simulink model "Tclab_simulink_model"  (R2021a)
settings: Solver=VariableStepAuto  StartTime=0.0  StopTime=600  RelTol=1e-3
undefined symbols (not defined in the file or in its folder): DiscIntNeverNeededParam, Discrete, ee_sli_rtmsupport, gcbh, Time
libraries: realtime_pacer_lib x2, sharedTrackingLibrary x1, ctrlSharedLib x1
settings Model: Creator=Arman  LastModifiedBy=Arman

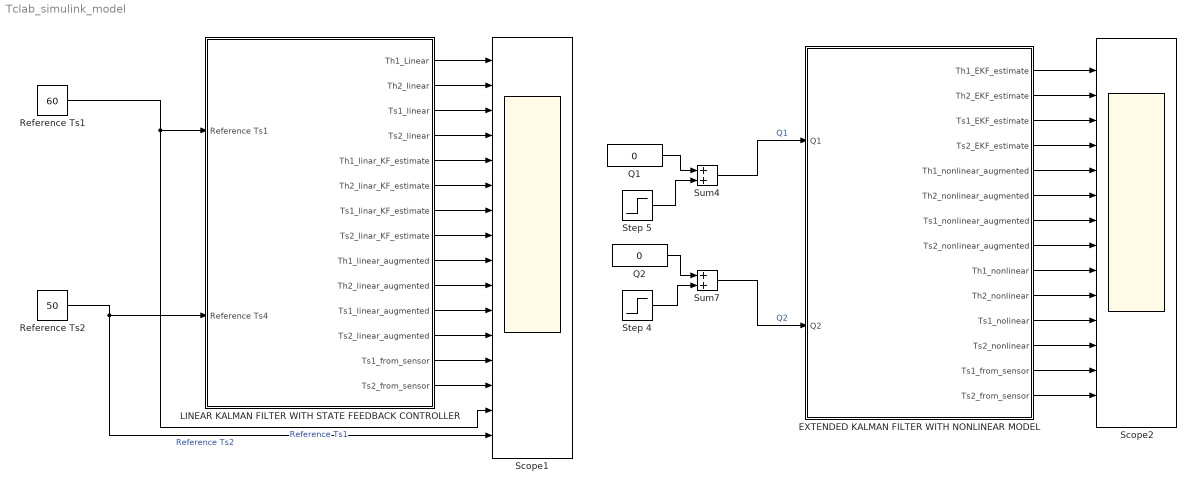
== system Tclab_simulink_model ==
  EXTENDED KALMAN FILTER WITH NONLINEAR MODEL : Subsystem
  LINEAR KALMAN FILTER WITH STATE FEEDBACK CONTROLLER : Subsystem
  Q1 : Constant  Value=0  SampleTime=1
  Q2 : Constant  Value=0  SampleTime=1
  "Reference Ts1 " : Constant  Value=60  SampleTime=1
  Reference Ts2 : Constant  Value=50  SampleTime=1
  Scope1 : Scope  NumInputPorts=16
  Scope2 : Scope  NumInputPorts=14
  Step 4 : Step  Time=300  Before=80  After=0  SampleTime=1
  Step 5 : Step  Time=300  After=80  SampleTime=1
  Sum4 : Sum  InputSameDT=on  SaturateOnIntegerOverflow=on  OutDataTypeStr=Inherit: Same as first input
  Sum7 : Sum  InputSameDT=on  SaturateOnIntegerOverflow=on  OutDataTypeStr=Inherit: Same as first input
  wires:
  "Reference Ts1 "/1 -> LINEAR KALMAN FILTER WITH STATE FEEDBACK CONTROLLER/1(Reference Ts1), Scope1/15  "Reference Ts1"
  Reference Ts2/1 -> Scope1/16, LINEAR KALMAN FILTER WITH STATE FEEDBACK CONTROLLER/2(Reference Ts4)  "Reference Ts2"
  Step 4/1 -> Sum7/2
  Q2/1 -> Sum7/1
  Step 5/1 -> Sum4/2
  Q1/1 -> Sum4/1
  Sum4/1 -> EXTENDED KALMAN FILTER WITH NONLINEAR MODEL/1(Q1)  "Q1"
  Sum7/1 -> EXTENDED KALMAN FILTER WITH NONLINEAR MODEL/2(Q2)  "Q2"
  LINEAR KALMAN FILTER WITH STATE FEEDBACK CONTROLLER/1(Th1_Linear) -> Scope1/1
  LINEAR KALMAN FILTER WITH STATE FEEDBACK CONTROLLER/2(Th2_linear) -> Scope1/2
  LINEAR KALMAN FILTER WITH STATE FEEDBACK CONTROLLER/3(Ts1_linear) -> Scope1/3
  LINEAR KALMAN FILTER WITH STATE FEEDBACK CONTROLLER/4(Ts2_linear) -> Scope1/4
  LINEAR KALMAN FILTER WITH STATE FEEDBACK CONTROLLER/5(Th1_linar_KF_estimate) -> Scope1/5
  LINEAR KALMAN FILTER WITH STATE FEEDBACK CONTROLLER/6(Th2_linar_KF_estimate) -> Scope1/6
  LINEAR KALMAN FILTER WITH STATE FEEDBACK CONTROLLER/7(Ts1_linar_KF_estimate) -> Scope1/7
  LINEAR KALMAN FILTER WITH STATE FEEDBACK CONTROLLER/8(Ts2_linar_KF_estimate) -> Scope1/8
  LINEAR KALMAN FILTER WITH STATE FEEDBACK CONTROLLER/9(Th1_linear_augmented) -> Scope1/9
  LINEAR KALMAN FILTER WITH STATE FEEDBACK CONTROLLER/10(Th2_linear_augmented) -> Scope1/10
  LINEAR KALMAN FILTER WITH STATE FEEDBACK CONTROLLER/11(Ts1_linear_augmented) -> Scope1/11
  LINEAR KALMAN FILTER WITH STATE FEEDBACK CONTROLLER/12(Ts2_linear_augmented) -> Scope1/12
  LINEAR KALMAN FILTER WITH STATE FEEDBACK CONTROLLER/13(Ts1_from_sensor) -> Scope1/13
  LINEAR KALMAN FILTER WITH STATE FEEDBACK CONTROLLER/14(Ts2_from_sensor) -> Scope1/14
  EXTENDED KALMAN FILTER WITH NONLINEAR MODEL/1(Th1_EKF_estimate) -> Scope2/1
  EXTENDED KALMAN FILTER WITH NONLINEAR MODEL/2(Th2_EKF_estimate) -> Scope2/2
  EXTENDED KALMAN FILTER WITH NONLINEAR MODEL/3(Ts1_EKF_estimate) -> Scope2/3
  EXTENDED KALMAN FILTER WITH NONLINEAR MODEL/4(Ts2_EKF_estimate) -> Scope2/4
  EXTENDED KALMAN FILTER WITH NONLINEAR MODEL/5(Th1_nonlinear_augmented) -> Scope2/5
  EXTENDED KALMAN FILTER WITH NONLINEAR MODEL/6(Th2_nonlinear_augmented) -> Scope2/6
  EXTENDED KALMAN FILTER WITH NONLINEAR MODEL/7(Ts1_nonlinear_augmented) -> Scope2/7
  EXTENDED KALMAN FILTER WITH NONLINEAR MODEL/8(Ts2_nonlinear_augmented) -> Scope2/8
  EXTENDED KALMAN FILTER WITH NONLINEAR MODEL/9(Th1_nonlinear) -> Scope2/9
  EXTENDED KALMAN FILTER WITH NONLINEAR MODEL/10(Th2_nonlinear) -> Scope2/10
  EXTENDED KALMAN FILTER WITH NONLINEAR MODEL/11(Ts1_nolinear) -> Scope2/11
  EXTENDED KALMAN FILTER WITH NONLINEAR MODEL/12(Ts2_nonlinear) -> Scope2/12
  EXTENDED KALMAN FILTER WITH NONLINEAR MODEL/13(Ts1_from_sensor) -> Scope2/13
  EXTENDED KALMAN FILTER WITH NONLINEAR MODEL/14(Ts2_from_sensor) -> Scope2/14

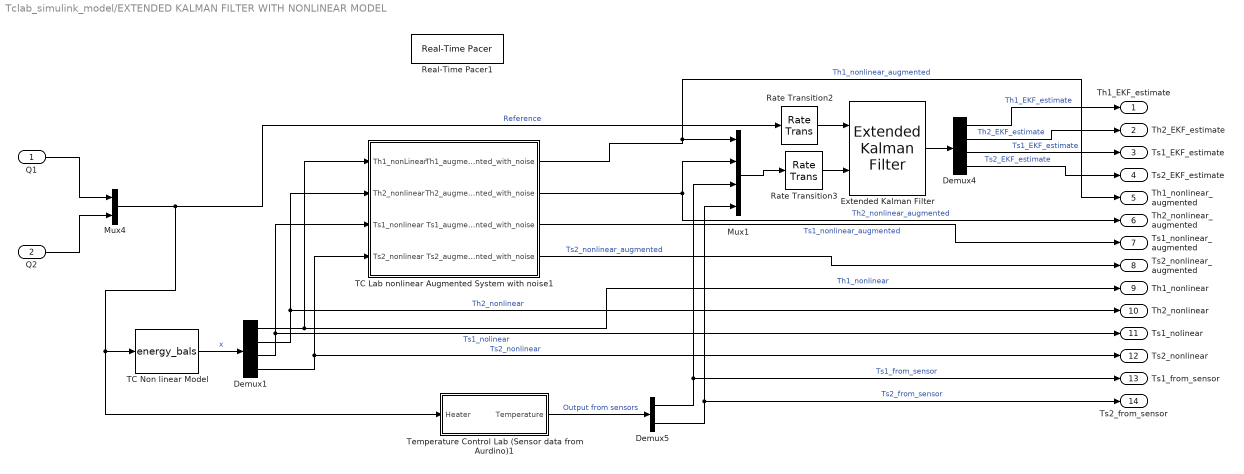
== system Tclab_simulink_model/EXTENDED KALMAN FILTER WITH NONLINEAR MODEL ==
  Q1 : Inport
  Q2 : Inport  Port=2
  Demux1 : Demux  Outputs=[1,1,1,1]
  Demux4 : Demux  Outputs=[1,1,1,1]
  Demux5 : Demux  Outputs=2
  Extended Kalman Filter : sharedTrackingLibrary/Extended Kalman Filter  StateTransitionFcn=myStateTransitionFcn  HasStateTransitionJacobianFcn=off  HasAdditiveProcessNoise=Additive  ProcessNoise=diag([1e-1 1e-1 1e-1 1e-1])  HasTimeVaryingProcessNoise=off  HasStateTransitionFcnExtraArgument=1  InitialState=[23 23 23 23]  InitialStateCovariance=diag([1e-6 1e-6 1e-6 1e-6 ])  MeasurementFcn1=myMeasurementFcn  HasMeasurementJacobianFcn1=off  HasMeasurementEnablePort1=off  HasAdditiveMeasurementNoise1=Additive  MeasurementNoise1=diag([1e-4 1e-4 1e-4 1e-4 ])  HasTimeVaryingMeasurementNoise1=off  HasMeasurementFcnExtraArgument1=0  MeasurementFcn2=myMeasurementFcn  HasMeasurementJacobianFcn2=off  HasMeasurementEnablePort2=off  HasAdditiveMeasurementNoise2=Additive  MeasurementNoise2=1  HasTimeVaryingMeasurementNoise2=off  HasMeasurementFcnExtraArgument2=0  MeasurementFcn3=myMeasurementFcn  HasMeasurementJacobianFcn3=off  HasMeasurementEnablePort3=off  HasAdditiveMeasurementNoise3=Additive  MeasurementNoise3=1  HasTimeVaryingMeasurementNoise3=off  HasMeasurementFcnExtraArgument3=0  MeasurementFcn4=myMeasurementFcn  HasMeasurementJacobianFcn4=off  HasMeasurementEnablePort4=off  HasAdditiveMeasurementNoise4=Additive  MeasurementNoise4=1  HasTimeVaryingMeasurementNoise4=off  HasMeasurementFcnExtraArgument4=0  MeasurementFcn5=myMeasurementFcn  HasMeasurementJacobianFcn5=off  HasMeasurementEnablePort5=off  HasAdditiveMeasurementNoise5=Additive  MeasurementNoise5=1  HasTimeVaryingMeasurementNoise5=off  HasMeasurementFcnExtraArgument5=0  EnableMultirate=off  StateTransitionFcnSampleTime=1  MeasurementFcn1SampleTime=1  MeasurementFcn2SampleTime=1  MeasurementFcn3SampleTime=1  MeasurementFcn4SampleTime=1  MeasurementFcn5SampleTime=1  UseCurrentEstimator=on  OutputStateCovariance=off  DataType=double  SampleTime=1  NumberOfMeasurements=1
      settings: SourceProductBaseCode=CT,DR,TF,ID,LP,NV,AR,RO,RR,UV,VE
  Mux1 : Mux
  Mux4 : Mux  Inputs=2
  Rate Transition2 : RateTransition  OutPortSampleTime=1
  Rate Transition3 : RateTransition  OutPortSampleTime=1
  Real-Time Pacer1 : realtime_pacer_lib/Real-Time Pacer  simTimePerRealTime=1
  TC Lab nonlinear Augmented System with noise1 : Subsystem
  "TC Non linear Model " : S-Function  FunctionName=energy_bals  SFunctionDeploymentMode=off  EnableBusSupport=off
  Temperature Control Lab (Sensor data from Aurdino)1 : Subsystem
  Th1_EKF_estimate : Outport
  Th2_EKF_estimate : Outport  Port=2
  Ts1_EKF_estimate : Outport  Port=3
  Ts2_EKF_estimate : Outport  Port=4
  Th1_nonlinear_augmented : Outport  Port=5
  Th2_nonlinear_augmented : Outport  Port=6
  Ts1_nonlinear_augmented : Outport  Port=7
  Ts2_nonlinear_augmented : Outport  Port=8
  Th1_nonlinear : Outport  Port=9
  Th2_nonlinear : Outport  Port=10
  Ts1_nolinear : Outport  Port=11
  Ts2_nonlinear : Outport  Port=12
  Ts1_from_sensor : Outport  Port=13
  Ts2_from_sensor : Outport  Port=14
  wires:
  Mux4/1 -> Rate Transition2/1, Temperature Control Lab (Sensor data from Aurdino)1/1(Heater), "TC Non linear Model "/1  "Reference"
  Rate Transition3/1 -> Extended Kalman Filter/2
  TC Lab nonlinear Augmented System with noise1/2(Th2_augmented_with_noise) -> Mux1/2, Th2_nonlinear_augmented/1  "Th2_nonlinear_augmented"
  Mux1/1 -> Rate Transition3/1
  Demux1/3 -> TC Lab nonlinear Augmented System with noise1/3(Ts1_nonlinear), Ts1_nolinear/1  "Ts1_nolinear"
  TC Lab nonlinear Augmented System with noise1/3(Ts1_augmented_with_noise) -> Ts1_nonlinear_augmented/1  "Ts1_nonlinear_augmented"
  Temperature Control Lab (Sensor data from Aurdino)1/1(Temperature) -> Demux5/1  "Output from sensors"
  Demux1/4 -> TC Lab nonlinear Augmented System with noise1/4(Ts2_nonlinear), Ts2_nonlinear/1  "Ts2_nonlinear"
  Rate Transition2/1 -> Extended Kalman Filter/1
  Extended Kalman Filter/1 -> Demux4/1
  "TC Non linear Model "/1 -> Demux1/1  "x"
  TC Lab nonlinear Augmented System with noise1/4(Ts2_augmented_with_noise) -> Ts2_nonlinear_augmented/1  "Ts2_nonlinear_augmented"
  Demux1/2 -> TC Lab nonlinear Augmented System with noise1/2(Th2_nonlinear), Th2_nonlinear/1  "Th2_nonlinear"
  Demux1/1 -> Th1_nonlinear/1, TC Lab nonlinear Augmented System with noise1/1(Th1_nonLinear)  "Th1_nonlinear"
  TC Lab nonlinear Augmented System with noise1/1(Th1_augmented_with_noise) -> Th1_nonlinear_augmented/1, Mux1/1  "Th1_nonlinear_augmented"
  Demux5/1 -> Mux1/3, Ts1_from_sensor/1  "Ts1_from_sensor"
  Q1/1 -> Mux4/1
  Q2/1 -> Mux4/2
  Demux5/2 -> Mux1/4, Ts2_from_sensor/1  "Ts2_from_sensor"
  Demux4/1 -> Th1_EKF_estimate/1  "Th1_EKF_estimate"
  Demux4/2 -> Th2_EKF_estimate/1  "Th2_EKF_estimate"
  Demux4/3 -> Ts1_EKF_estimate/1  "Ts1_EKF_estimate"
  Demux4/4 -> Ts2_EKF_estimate/1  "Ts2_EKF_estimate"

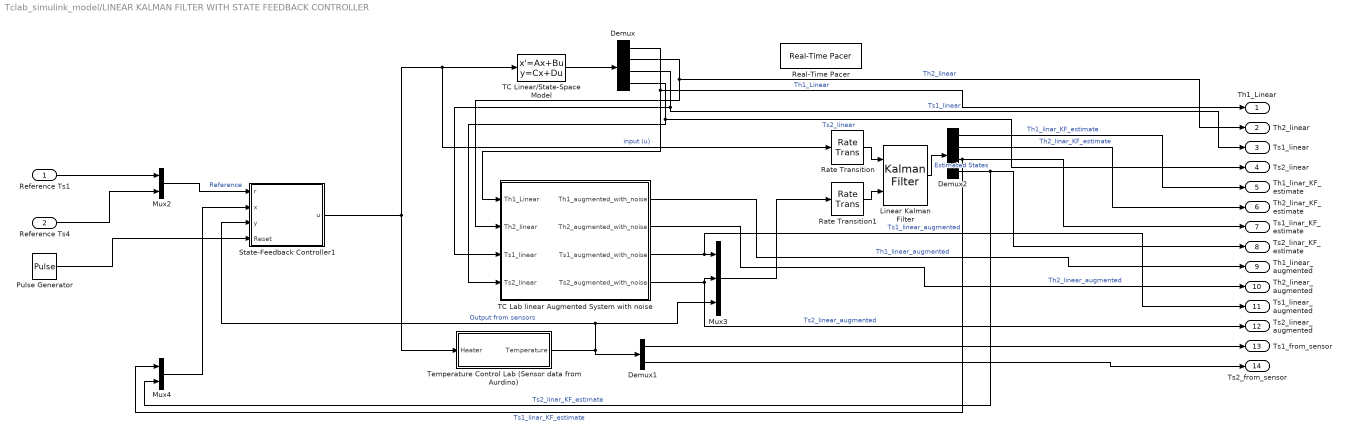
== system Tclab_simulink_model/LINEAR KALMAN FILTER WITH STATE FEEDBACK CONTROLLER ==
  Reference Ts1 : Inport
  Reference Ts4 : Inport  Port=2
  Demux : Demux  Outputs=[1,1,1,1]
  Demux1 : Demux  Outputs=2
  Demux2 : Demux  Outputs=[1,1,1,1]
  Linear Kalman Filter : ctrlSharedLib/Kalman Filter  TimeDomain=Discrete-Time  UseCurrentEstimator=on  ModelSource=Individual A, B, C, D matrices  ModelSourceVariable=linsys1  A=[-0.007 0.002 0 0; 0.002 -0.007 0 0; 0.050 0 -0.050 0; 0 0.050 0 -0.050]  B=[0.005 0; 0 0.0038; 0 0; 0 0]  C=diag([1 1 1 1])  D=zeros(4,2)  NumberOfStates=2  NumberOfInputs=2  NumberOfOutputs=2  InitialEstimateSource=Dialog  X0=[23 23 23 23]  P0=10  UseK=off  UseGH=off  NumberOfProcessNoiseInputs=1  G=[0; 0; 0; 0]  TimeInvariantG=on  H=[20; 20; 20; 20]  TimeInvariantH=on  Q=10  TimeInvariantQ=on  R=10/50  TimeInvariantR=on  N=0  TimeInvariantN=on  AddInputPort=on  AddEnablePort=off  OutputEstimatedY=off  OutputP=off  Ts=1
  Mux2 : Mux  Inputs=2
  Mux3 : Mux  Inputs=3
  Mux4 : Mux  Inputs=2
  Pulse Generator : DiscretePulseGenerator  PulseType=Time based  Period=1  PulseWidth=50
  Rate Transition : RateTransition  OutPortSampleTime=1
  Rate Transition1 : RateTransition  OutPortSampleTime=1
  Real-Time Pacer : realtime_pacer_lib/Real-Time Pacer  simTimePerRealTime=1
  State-Feedback Controller1 : Subsystem  AncestorBlock=eeAlternativeControllers/State-Feedback Controller  LoadFcn=ee_sli_rtmsupport( 'loadfcn', gcbh );  mask(State-Feedback Controller){StateFeedbackDesign=State-feedback gain, StateSpaceType=Discrete-time, K=lqr([-0.007 0.002 0 0; 0.002 -0.007 0 0; 0.050 0 -0.050 0; 0 0.050 0 -0.050],[0.005 0; 0 0.0038; 0 0; 0 0],.07,1,0), Ad=1, Bd=1, Cd=1, Dd=0, A=1, B=1, C=1, D=0, Tsd=0.1, DesiredEigenvalues=[0.5 0.6], up=80, lo=30, Ts=-1}
      mask prompts: StateFeedbackDesign "physmod:ee:library:comments:control:eeAlternativeControllers:StatefeedbackDesign_MP"; StateSpaceType "physmod:ee:library:comments:control:eeAlternativeControllers:StatefeedbackParameterization_MP"; K "physmod:ee:library:comments:control:eeAlternativeControllers:ControllerMatrix_MP"; Ad "physmod:ee:library:comments:control:eeAlternativeControllers:DiscretetimeAMatrix_MP"; Bd "physmod:ee:library:comments:control:eeAlternativeControllers:DiscretetimeBMatrix_MP"; Cd "physmod:ee:library:comments:control:eeAlternativeControllers:DiscretetimeCMatrix_MP"; Dd "physmod:ee:library:comments:control:eeAlternativeControllers:DiscretetimeDMatrix_MP"; A "physmod:ee:library:comments:control:eeAlternativeControllers:ContinuoustimeAMatrix_MP"; B "physmod:ee:library:comments:control:eeAlternativeControllers:ContinuoustimeBMatrix_MP"; C "physmod:ee:library:comments:control:eeAlternativeControllers:ContinuoustimeCMatrix_MP"; D "physmod:ee:library:comments:control:eeAlternativeControllers:ContinuoustimeDMatrix_MP"; Tsd "physmod:ee:library:comments:control:eeAlternativeControllers:DiscretizationSampleTime_MP"; DesiredEigenvalues "physmod:ee:library:comments:control:eeAlternativeControllers:DesiredEigenvaluesdiscrete_MP"; up "physmod:ee:library:comments:control:eeAlternativeControllers:ControlActionUpperLimit_MP"; lo "physmod:ee:library:comments:control:eeAlternativeControllers:ControlActionLowerLimit_MP"; Ts "physmod:ee:library:comments:control:eeAlternativeControllers:SampleTime1ForInherited_MP"
      mask help: physmod:ee:library:comments:control:eeAlternativeControllers:StateFeedbackController_MD
      mask init:
      | K = ee.mask.initializeStateFeedbackController(StateFeedbackDesign, StateSpaceType, K, Ad, Bd, Cd, Dd, A, B, C, D, DesiredEigenvalues, up, lo, Ts, Tsd);
      settings: CopyFcn=ee_sli_rtmsupport( 'copyfcn', gcbh );  DeleteFcn=ee_sli_rtmsupport( 'deletefcn', gcbh );  ModelCloseFcn=ee_sli_rtmsupport( 'modelclosefcn', gcbh );  PostSaveFcn=ee_sli_rtmsupport( 'postsavefcn', gcbh );  PreCopyFcn=ee_sli_rtmsupport( 'precopyfcn', gcbh );  OpenFcn=ee_sli_rtmsupport( 'openfcn', gcbh );  CloseFcn=ee_sli_rtmsupport( 'closefcn', gcbh );  PreDeleteFcn=ee_sli_rtmsupport( 'predeletefcn', gcbh );
      mask Help: web(nesl_help(gcbh))
      mask TypeOptions StateFeedbackDesign: physmod:ee:library:comments:control:eeAlternativeControllers:State0x2DFeedbackGain_PV | physmod:ee:library:comments:control:eeAlternativeControllers:DesiredEigenvalues_PV
      mask Callback StateFeedbackDesign: ee.mask.callbackStateFeedbackController(gcb)
      mask TypeOptions StateSpaceType: physmod:ee:library:comments:control:eeAlternativeControllers:Discrete0x2DTime_PV | physmod:ee:library:comments:control:eeAlternativeControllers:Continuous0x2DTime_PV
      mask Callback StateSpaceType: ee.mask.callbackStateFeedbackController(gcb)
      mask Callback B: ee.mask.callbackStateFeedbackController(gcb)
      mask Callback Ts: ee.mask.callbackStateFeedbackController(gcb)
      mask DialogControl StateFeedbackDesign Prompt: State-feedback design
      mask DialogControl StateSpaceType Prompt: State-feedback parameterization
      mask DialogControl K Prompt: Controller matrix
      mask DialogControl Ad Prompt: Discrete-time A matrix
      mask DialogControl Bd Prompt: Discrete-time B matrix
      mask DialogControl Cd Prompt: Discrete-time C matrix
      mask DialogControl Dd Prompt: Discrete-time D matrix
      mask DialogControl A Prompt: Continuous-time A matrix
      mask DialogControl B Prompt: Continuous-time B matrix
      mask DialogControl C Prompt: Continuous-time C matrix
      mask DialogControl D Prompt: Continuous-time D matrix
      mask DialogControl Tsd Prompt: Discretization sample time
      mask DialogControl DesiredEigenvalues Prompt: Desired eigenvalues (discrete)
      mask DialogControl up Prompt: Control action upper limit
      mask DialogControl lo Prompt: Control action lower limit
      mask DialogControl Ts Prompt: Sample time (-1 for inherited)
  TC Lab linear Augmented System with noise : Subsystem
  TC Linear/State-Space Model : StateSpace  A=[-0.007 0.002 0 0; 0.002 -0.007 0 0; 0.050 0 -0.050 0; 0 0.050 0 -0.050]  B=[0.005 0; 0 0.0038; 0 0; 0 0]  C=diag([1 1 1 1])  D=zeros(4,2)  InitialCondition=[23 23 23 23]
  Temperature Control Lab (Sensor data from Aurdino) : Subsystem
  Th1_Linear : Outport
  Th2_linear : Outport  Port=2
  Ts1_linear : Outport  Port=3
  Ts2_linear : Outport  Port=4
  Th1_linar_KF_estimate : Outport  Port=5
  Th2_linar_KF_estimate : Outport  Port=6
  Ts1_linar_KF_estimate : Outport  Port=7
  Ts2_linar_KF_estimate : Outport  Port=8
  Th1_linear_augmented : Outport  Port=9
  Th2_linear_augmented : Outport  Port=10
  Ts1_linear_augmented : Outport  Port=11
  Ts2_linear_augmented : Outport  Port=12
  Ts1_from_sensor : Outport  Port=13
  Ts2_from_sensor : Outport  Port=14
  wires:
  TC Lab linear Augmented System with noise/3(Ts1_augmented_with_noise) -> Ts1_linear_augmented/1, Mux3/1  "Ts1_linear_augmented"
  TC Lab linear Augmented System with noise/4(Ts2_augmented_with_noise) -> Ts2_linear_augmented/1, Mux3/2  "Ts2_linear_augmented"
  Linear Kalman Filter/1 -> Demux2/1  "Estimated States"
  Rate Transition1/1 -> Linear Kalman Filter/2
  Rate Transition/1 -> Linear Kalman Filter/1
  Demux/4 -> Ts2_linear/1, TC Lab linear Augmented System with noise/4(Ts2_linear)  "Ts2_linear"
  Demux/3 -> Ts1_linear/1, TC Lab linear Augmented System with noise/3(Ts1_linear)  "Ts1_linear"
  Reference Ts1/1 -> Mux2/1
  Demux2/2 -> Th2_linar_KF_estimate/1  "Th2_linar_KF_estimate"
  TC Lab linear Augmented System with noise/1(Th1_augmented_with_noise) -> Th1_linear_augmented/1  "Th1_linear_augmented"
  Mux3/1 -> Rate Transition1/1
  Demux/2 -> Th2_linear/1, TC Lab linear Augmented System with noise/2(Th2_linear)  "Th2_linear"
  State-Feedback Controller1/1(u) -> Temperature Control Lab (Sensor data from Aurdino)/1(Heater), TC Linear/State-Space Model/1, Rate Transition/1  "input (u)"
  Mux2/1 -> State-Feedback Controller1/1(r)  "Reference"
  TC Linear/State-Space Model/1 -> Demux/1
  Demux2/1 -> Th1_linar_KF_estimate/1  "Th1_linar_KF_estimate"
  Reference Ts4/1 -> Mux2/2
  Demux/1 -> Th1_Linear/1, TC Lab linear Augmented System with noise/1(Th1_Linear)  "Th1_Linear"
  Demux2/4 -> Mux4/2, Ts2_linar_KF_estimate/1  "Ts2_linar_KF_estimate"
  Demux2/3 -> Mux4/1, Ts1_linar_KF_estimate/1  "Ts1_linar_KF_estimate"
  TC Lab linear Augmented System with noise/2(Th2_augmented_with_noise) -> Th2_linear_augmented/1  "Th2_linear_augmented"
  Pulse Generator/1 -> State-Feedback Controller1/4(Reset)
  Mux4/1 -> State-Feedback Controller1/2(x)
  Demux1/1 -> Ts1_from_sensor/1
  Demux1/2 -> Ts2_from_sensor/1
  Temperature Control Lab (Sensor data from Aurdino)/1(Temperature) -> State-Feedback Controller1/3(y), Mux3/3, Demux1/1  "Output from sensors"

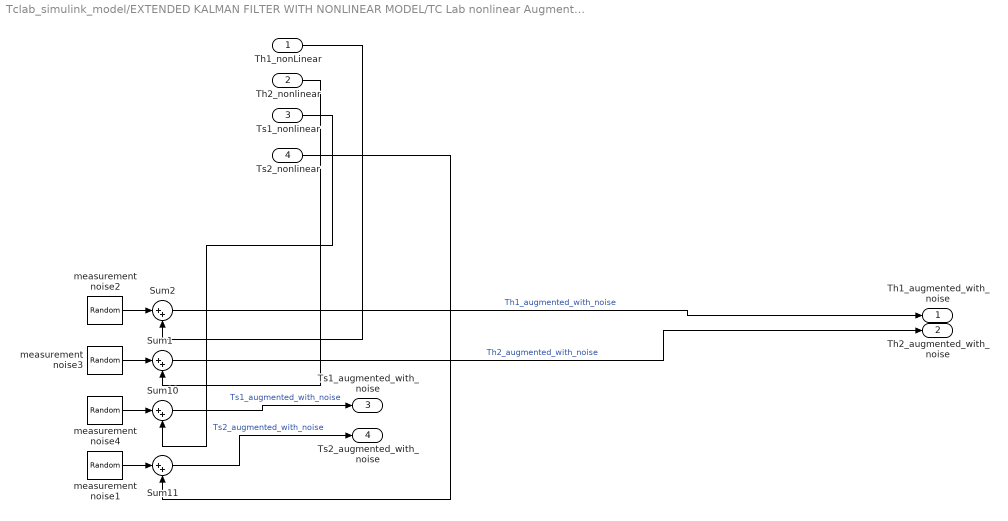
== system Tclab_simulink_model/EXTENDED KALMAN FILTER WITH NONLINEAR MODEL/TC Lab nonlinear Augmented System with noise1 ==
  Th1_nonLinear : Inport
  Th2_nonlinear : Inport  Port=2
  Ts1_nonlinear : Inport  Port=3
  Ts2_nonlinear : Inport  Port=4
  Sum{1..2,10..11} (4 alike) : Sum  Inputs=|++
  measurement noise{1..4} (4 alike) : RandomNumber  Variance=1e-2  SampleTime=1
  Th1_augmented_with_noise : Outport
  Th2_augmented_with_noise : Outport  Port=2
  Ts1_augmented_with_noise : Outport  Port=3
  Ts2_augmented_with_noise : Outport  Port=4
  wires:
  Sum10/1 -> Ts1_augmented_with_noise/1  "Ts1_augmented_with_noise"
  measurement noise3/1 -> Sum1/1
  measurement noise2/1 -> Sum2/1
  measurement noise4/1 -> Sum10/1
  measurement noise1/1 -> Sum11/1
  Sum2/1 -> Th1_augmented_with_noise/1  "Th1_augmented_with_noise"
  Ts1_nonlinear/1 -> Sum10/2
  Th1_nonLinear/1 -> Sum2/2
  Sum11/1 -> Ts2_augmented_with_noise/1  "Ts2_augmented_with_noise"
  Ts2_nonlinear/1 -> Sum11/2
  Th2_nonlinear/1 -> Sum1/2
  Sum1/1 -> Th2_augmented_with_noise/1  "Th2_augmented_with_noise"

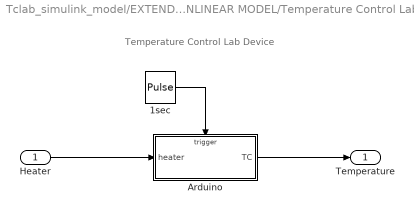
== system Tclab_simulink_model/EXTENDED KALMAN FILTER WITH NONLINEAR MODEL/Temperature Control Lab (Sensor data from Aurdino)1 ==
  note: Temperature Control Lab Device
  Heater : Inport
  1sec : DiscretePulseGenerator  PulseType=Time based  Period=1  PulseWidth=50
  Arduino : Subsystem  TreatAsAtomicUnit=on
  Temperature : Outport  VectorParamsAs1DForOutWhenUnconnected=off
  wires:
  1sec/1 -> Arduino/Trigger
  Arduino/1(TC) -> Temperature/1
  Heater/1 -> Arduino/1(heater)

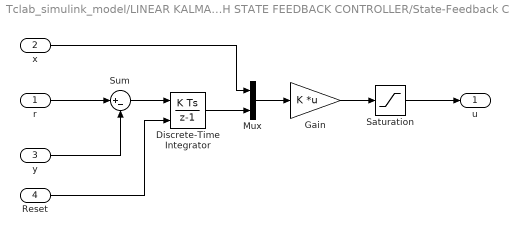
== system Tclab_simulink_model/LINEAR KALMAN FILTER WITH STATE FEEDBACK CONTROLLER/State-Feedback Controller1 ==
  r : Inport  SampleTime=Ts
  x : Inport  Port=2  SampleTime=Ts
  y : Inport  Port=3  SampleTime=Ts
  Reset : Inport  Port=4  SampleTime=Ts
  Discrete-Time Integrator : DiscreteIntegrator  gainval=1  ExternalReset=rising  SampleTime=Ts  ICPrevOutput=DiscIntNeverNeededParam  ICPrevScaledInput=DiscIntNeverNeededParam
  Gain : Gain  Gain=K  Multiplication=Matrix(K*u)
  Mux : Mux  Inputs=2
  Saturation : Saturate  UpperLimit=up  LowerLimit=lo
  Sum : Sum  Inputs=|+-
  u : Outport  VectorParamsAs1DForOutWhenUnconnected=off
  wires:
  Sum/1 -> Discrete-Time Integrator/1
  x/1 -> Mux/1
  Discrete-Time Integrator/1 -> Mux/2
  Mux/1 -> Gain/1
  Gain/1 -> Saturation/1
  r/1 -> Sum/1
  y/1 -> Sum/2
  Saturation/1 -> u/1
  Reset/1 -> Discrete-Time Integrator/2

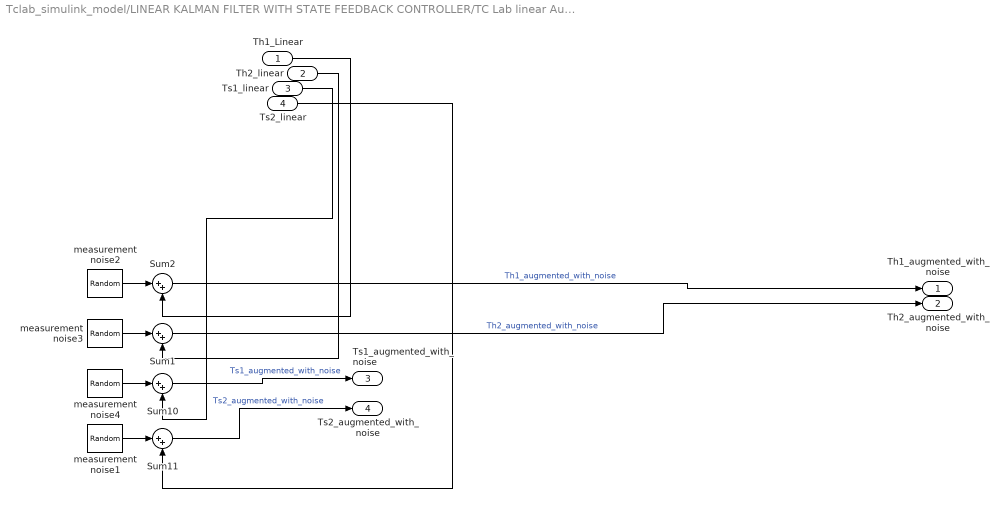
== system Tclab_simulink_model/LINEAR KALMAN FILTER WITH STATE FEEDBACK CONTROLLER/TC Lab linear Augmented System with noise ==
  Th1_Linear : Inport
  Th2_linear : Inport  Port=2
  Ts1_linear : Inport  Port=3
  Ts2_linear : Inport  Port=4
  Sum{1..2,10..11} (4 alike) : Sum  Inputs=|++
  measurement noise{1..4} (4 alike) : RandomNumber  Variance=1e-1  SampleTime=1
  Th1_augmented_with_noise : Outport
  Th2_augmented_with_noise : Outport  Port=2
  Ts1_augmented_with_noise : Outport  Port=3
  Ts2_augmented_with_noise : Outport  Port=4
  wires:
  Sum10/1 -> Ts1_augmented_with_noise/1  "Ts1_augmented_with_noise"
  measurement noise3/1 -> Sum1/1
  measurement noise2/1 -> Sum2/1
  measurement noise4/1 -> Sum10/1
  measurement noise1/1 -> Sum11/1
  Sum2/1 -> Th1_augmented_with_noise/1  "Th1_augmented_with_noise"
  Ts1_linear/1 -> Sum10/2
  Th1_Linear/1 -> Sum2/2
  Sum11/1 -> Ts2_augmented_with_noise/1  "Ts2_augmented_with_noise"
  Ts2_linear/1 -> Sum11/2
  Th2_linear/1 -> Sum1/2
  Sum1/1 -> Th2_augmented_with_noise/1  "Th2_augmented_with_noise"

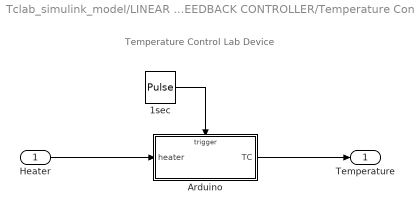
== system Tclab_simulink_model/LINEAR KALMAN FILTER WITH STATE FEEDBACK CONTROLLER/Temperature Control Lab (Sensor data from Aurdino) ==
  note: Temperature Control Lab Device
  Heater : Inport
  1sec : DiscretePulseGenerator  PulseType=Time based  Period=1  PulseWidth=50
  Arduino : Subsystem  TreatAsAtomicUnit=on
  Temperature : Outport  VectorParamsAs1DForOutWhenUnconnected=off
  wires:
  1sec/1 -> Arduino/Trigger
  Arduino/1(TC) -> Temperature/1
  Heater/1 -> Arduino/1(heater)

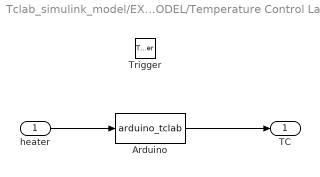
== system Tclab_simulink_model/EXTENDED KALMAN FILTER WITH NONLINEAR MODEL/Temperature Control Lab (Sensor data from Aurdino)1/Arduino ==
  heater : Inport  LatchByDelayingOutsideSignal=on
  Trigger : TriggerPort  VariantControl=Variant
  Arduino : MATLABFcn  MATLABFcn=arduino_tclab
  TC : Outport  InitialOutput=23  VectorParamsAs1DForOutWhenUnconnected=off
  wires:
  heater/1 -> Arduino/1
  Arduino/1 -> TC/1

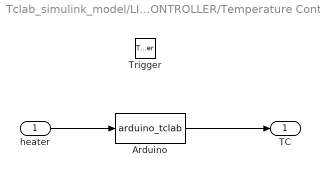
== system Tclab_simulink_model/LINEAR KALMAN FILTER WITH STATE FEEDBACK CONTROLLER/Temperature Control Lab (Sensor data from Aurdino)/Arduino ==
  heater : Inport  LatchByDelayingOutsideSignal=on
  Trigger : TriggerPort  VariantControl=Variant
  Arduino : MATLABFcn  MATLABFcn=arduino_tclab
  TC : Outport  InitialOutput=23  VectorParamsAs1DForOutWhenUnconnected=off
  wires:
  heater/1 -> Arduino/1
  Arduino/1 -> TC/1
